simulink model "x64_15l_gonly"  (R2012b)
settings: Solver=VariableStepDiscrete  SolverMode=SingleTasking  StartTime=0.0  StopTime=10.0  RelTol=1e-3
undefined symbols (not defined in the file): gcbh, pfb_coeff_gen_calc, ROACH, xlBlockLoadCallback
libraries: xbsIndex_r4 x10760, casper_library_misc x122, casper_library_delays x52, ox_lib x14, xrbsComm_r4 x8, xps_library x8
(part 4 of 128)

== system x64_15l_gonly/chan_reorder ==
  sync : Inport
  din : Inport  Port=2
  Constant : xbsIndex_r4/Constant  const=1  gui_display_data_type=Fixed-point  arith_type=Boolean  n_bits=16  bin_pt=14  preci_type=Single  exp_width=8  frac_width=24  explicit_period=on  period=1  equ=P=C  opselect=C  inp2=PCIN>>17  opr=+  inp1=P  carry=CIN  dbl_ovrd=off  block_type=constant
      settings: block_version=11.4
  reorder : Subsystem  AncestorBlock=casper_library_reorder/reorder  mask(reorder){map=[0                                    512                                      1                                    513                                      2                                    514                                      3                                    515                                      4                                    516                                      5                                    517                                      6                                    518                                      7                                    519                                      8                                    520                                      9                                    521                                     10                                    522                                     11                                    523                                     12                                    524                                     13                                    525                                     14                                    526                                     15                                    527                                     16                                    528                                     17                                    529                                     18                                    530                                     19                                    531                                     20                                    532                                     21                                    533                                     22                                    534                                     23                                    535                                     24                                    536                                     25                                    537                                     26                                    538                                     27                                    539                                     28                                    540                                     29                                    541                                     30                                    542                                     31                                    543                                     32                                    544                                     33                                    545                                     34                                    546                                     35                                    547                                     36                                    548                                     37                                    549                                     38                                    550                                     39                                    551                                     40                                    552                                     41                                    553                                     42                                    554                                     43                                    555                                     44                                    556                                     45                                    557                                     46                                    558                                     47                                    559                                     48                                    560                                     49                                    561                                     50                                    562                                     51 ...(+35900 chars)], n_bits=0, n_inputs=1, bram_latency=2, map_latency=0, fanout_latency=0, double_buffer=0, bram_map=off}
      mask prompts: map "Output Order:"; n_bits "Data width in"; n_inputs "Number of inputs"; bram_latency "BRAM Latency"; map_latency "Map Latency"; fanout_latency "Fanout latency"; double_buffer "Double Buffer"; bram_map "Use BlockRAM for Map"
      mask init: same as x64_15l_gonly/reorder
      settings: AttributesFormatString=order=10
      mask Help: eval('xlWeb(''http://casper.berkeley.edu/wiki/Reorder'')')
  sync_out : Outport
  dout : Outport  Port=2
  wires:
  reorder/3(dout0) -> dout/1
  din/1 -> reorder/3(din0)
  Constant/1 -> reorder/2(en)
  reorder/1(sync_out) -> sync_out/1
  sync/1 -> reorder/1(sync)

== system x64_15l_gonly/ctrl_sw ==
  sim_1 : Inport
  io_delay : xbsIndex_r4/Delay  rst=off  infoeditControl=Selection of Reset will increase slice count due to use of real FFs and instead of SRLs  en=off  latency=0  dbl_ovrd=off  reg_retiming=on  block_type=delay
  reint1 : xbsIndex_r4/Reinterpret  force_arith_type=on  arith_type=Unsigned  force_bin_pt=on  bin_pt=0  block_type=reinterpret
  slice_reg : xbsIndex_r4/Slice  nbits=32  boolean_output=off  mode=Lower Bit Location + Width  bit1=0  base1=MSB of Input  bit0=0  base0=LSB of Input  dbl_ovrd=off  block_type=slice
  x64_32f_2014_ctrl_sw_user_data_out : xbsIndex_r4/Gateway In  gui_display_data_type=Fixed-point  arith_type=Unsigned  n_bits=32  bin_pt=0  preci_type=Single  exp_width=8  frac_width=24  quantization="Round  (unbiased: +/- Inf)"  overflow=Saturate  period=1  dbl_ovrd=off  timing_constraint=None  locs_specified=off  LOCs={}  UseAsADC=off  ADCChannel='1'  inherit_from_input=off  hdl_port=on  block_type=gatewayin
  in_reg : Outport
  wires:
  x64_32f_2014_ctrl_sw_user_data_out/1 -> io_delay/1
  sim_1/1 -> x64_32f_2014_ctrl_sw_user_data_out/1
  io_delay/1 -> slice_reg/1
  slice_reg/1 -> reint1/1
  reint1/1 -> in_reg/1

== system x64_15l_gonly/edge_detect ==
  in : Inport
  Delay : xbsIndex_r4/Delay  rst=off  infoeditControl=Selection of Reset will increase slice count due to use of real FFs and instead of SRLs  en=off  latency=1  dbl_ovrd=off  reg_retiming=off  block_type=delay
      settings: xl_area=[0, 0, 0, 0, 0, 0, 0]
  Inverter : xbsIndex_r4/Inverter  en=off  latency=0  dbl_ovrd=off  block_type=inv
      settings: xl_area=[0, 0, 0, 0, 0, 0, 0]
  edge_op : xbsIndex_r4/Logical  logical_function=NOR  inputs=2  en=off  latency=0  precision=Full  arith_type=Unsigned  n_bits=8  bin_pt=2  align_bp=on  dbl_ovrd=off  block_type=logical
      settings: xl_area=[0, 0, 0, 0, 0, 0, 0]
  out : Outport
  wires:
  Inverter/1 -> edge_op/1
  edge_op/1 -> out/1
  in/1 -> Inverter/1, Delay/1
  Delay/1 -> edge_op/2
